simulink model "roboSubDetectWithObjectDetectorBlock"  (R2022b)
settings: Solver=VariableStepAuto  StartTime=0.0  StopTime=10.0  RelTol=1e-3
libraries: visionanalysis x1, dspvision x1
settings Model: Creator=gracew  LastModifiedBy=gracew
settings SFSimCC: SimTargetLang=C++

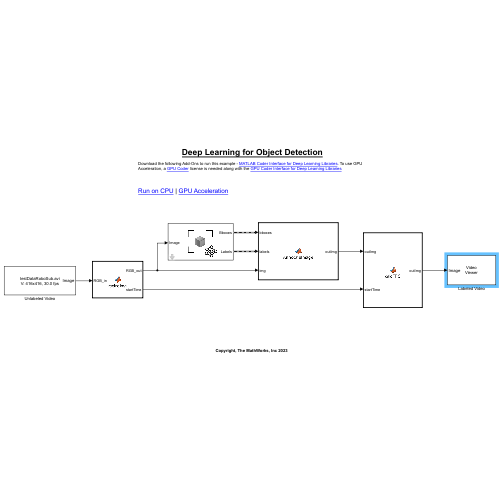
[thumbnail: Simulink's stored preview of the top-level diagram]
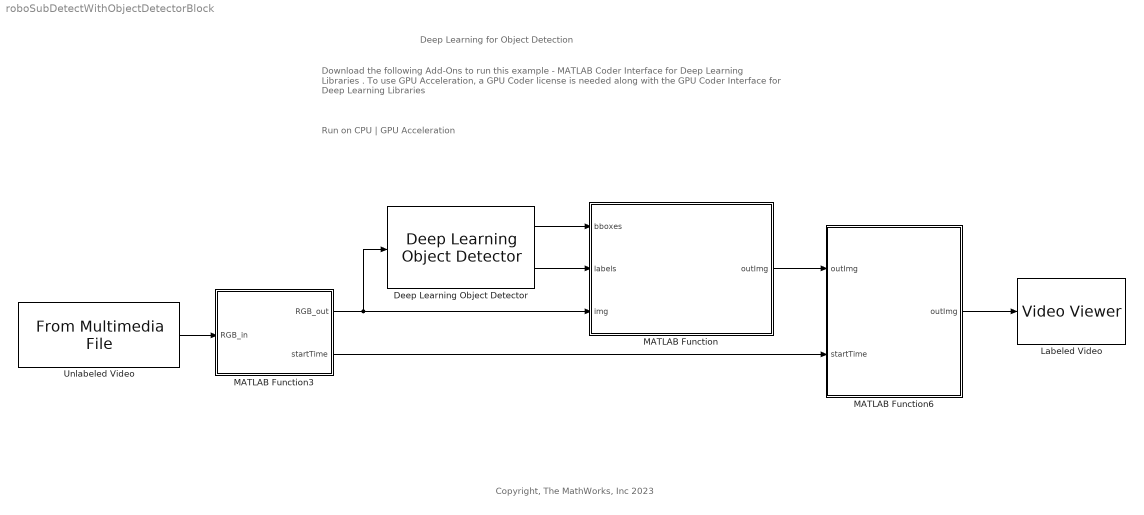
== system roboSubDetectWithObjectDetectorBlock ==
  note: Deep Learning for Object Detection
  note: Run on CPU | GPU Acceleration
  note: Download the following Add-Ons to run this example - MATLAB Coder Interface for Deep Learning Libraries . To use GPU Acceleration, a GPU Coder license is needed along with the GPU Coder Interface for Deep Learning Libraries
  note: Copyright, The MathWorks, Inc 2023
  Deep Learning Object Detector : visionanalysis/Deep Learning Object Detector  Detector=Detector from MAT-file  DetectorFunction=untitled  DetectorFilePath=detectorYoloV2.mat  MaxDetections=500  Bboxes=on  Scores=off  UseROI=off  ROI=[1 1 100 100]  Threshold=0.5  NumStrongestRegions=2000  UseMinSize=off  MinSize=[1 1]  UseMaxSize=off  MaxSize=[50 50]  ForceInterpretedSim=off
  Labeled Video : VideoViewer  FigPos=[502.333333333333 621.333333333333 440 360]
  MATLAB Function : MATLAB Function  TreatAsAtomicUnit=on
  MATLAB Function3 : MATLAB Function  TreatAsAtomicUnit=on
  MATLAB Function6 : MATLAB Function  TreatAsAtomicUnit=on
  Unlabeled Video : dspvision/From Multimedia File  inputFilename=testDataRoboSub.avi  readRange=[1 Inf]  loop=on  numPlays=inf  outputStreams=Video only  videoDataType=single  audioDataType=int16  inheritSampleTime=on  userDefinedSampleTime=1/30  noAudioOutput=off  isIntensityVideo=off  fourcc=RGB  colorVideoFormat=One multidimensional signal  outputEOF=off  dataOrg=Column-major  audioFrameSize=1024  computeAudioFrameSize=off  outSamplingMode=Sample based
  wires:
  Deep Learning Object Detector/1 -> MATLAB Function/1(bboxes)
  MATLAB Function3/1(RGB_out) -> MATLAB Function/3(img), Deep Learning Object Detector/1
  Deep Learning Object Detector/2 -> MATLAB Function/2(labels)
  MATLAB Function/1(outImg) -> MATLAB Function6/1("outImg ")
  MATLAB Function3/2(startTime) -> MATLAB Function6/2(startTime)
  MATLAB Function6/1(outImg) -> Labeled Video/1
  Unlabeled Video/1 -> MATLAB Function3/1(RGB_in)

== matlab function roboSubDetectWithObjectDetectorBlock/MATLAB Function ==
  data: bboxes input; labels input; outImg output; img input
function outImg = AnnotateImage(bboxes, labels, img)
    % Annotate detections in the image. 

    if ~isempty(bboxes)
        for i = 1:numel(labels)
            img = insertObjectAnnotation(img, "rectangle", bboxes(i, :), char(labels(i)));
        end
    end

    outImg = img;

end

== matlab function roboSubDetectWithObjectDetectorBlock/MATLAB Function3 ==
  data: RGB_in input; RGB_out output; startTime output
function [RGB_out, startTime] = resizeImg(RGB_in)
    RGB_out = imresize(RGB_in,[416,416]);
    
    currentTime = datetime;
    startTime = [currentTime.Year currentTime.Month currentTime.Day currentTime.Hour ...
        currentTime.Minute currentTime.Second];
end

== matlab function roboSubDetectWithObjectDetectorBlock/MATLAB Function6 ==
  data: outImg input; startTime input; outImg output
function outImg  = calcFPS(outImg, startTime)
    finishTime = datetime;
    
    diffTime = seconds(finishTime-datetime(startTime));
    persistent count;
    if isempty(count)
        count = 0;
    end
    persistent fps;
    if isempty(fps)
        fps = 0;
    end
    fps = (count*fps + 1*(1/diffTime))/(count+1);
    
    count = count + 1;
    outImg = insertText(outImg, [10 80],['FPS : ' sprintf('%0.2f',fps) ], 'AnchorPoint','LeftBottom');
end
